simulink model "AOM"  (R2023a)
settings: Solver=ode4  StartTime=0.0  StopTime=4  FixedStep=0.001  RelTol=1e-3
values from neighbouring files (symbols this model uses):
  trajectory = readmatrix('test.csv')    [actor_critic.m]
undefined symbols (not defined in the file or in its folder): dot_X0, X0
libraries: rllib x1
settings Model: Creator=Ali  LastModifiedBy=Ali

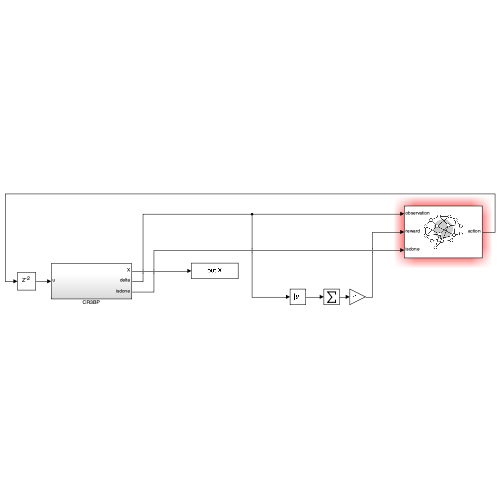
[thumbnail: Simulink's stored preview of the top-level diagram]
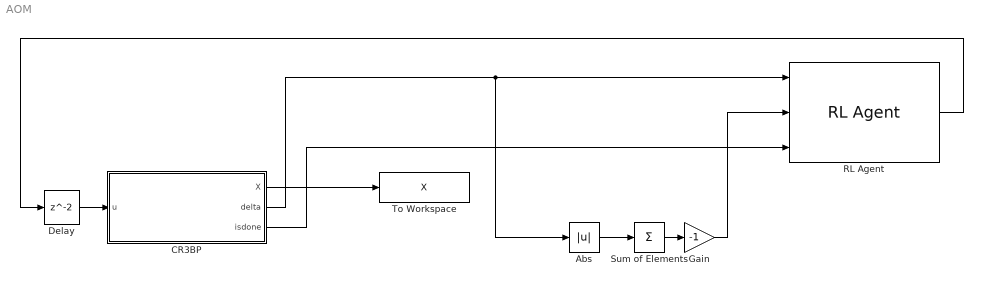
== system AOM ==
  Abs : Abs  SaturateOnIntegerOverflow=off
  CR3BP : Subsystem
  Delay : Delay
  Gain : Gain  Gain=-1
  RL Agent : rllib/RL Agent  Agent=agentObj  ExternalActionAsInput=off  ProvideLastAction=off  ProvideCumRwd=off  TreatAsDirectFeedthrough=on  UseStrictObservationDataTypes=off
  Sum of Elements : Sum  Inputs=+
  To Workspace : ToWorkspace  VariableName=X  SaveFormat=Timeseries  SampleTime=-1
  wires:
  CR3BP/1(X) -> To Workspace/1
  CR3BP/3(isdone) -> RL Agent/3
  RL Agent/1 -> Delay/1
  Delay/1 -> CR3BP/1(u)
  CR3BP/2(delta) -> Abs/1, RL Agent/1
  Abs/1 -> Sum of Elements/1
  Sum of Elements/1 -> Gain/1
  Gain/1 -> RL Agent/2

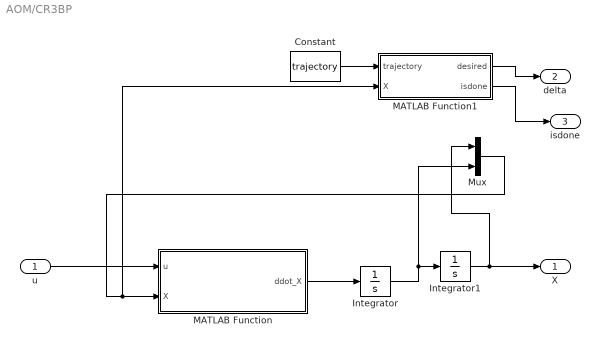
== system AOM/CR3BP ==
  u : Inport
  Constant : Constant  Value=trajectory
  Integrator : Integrator  InitialCondition=dot_X0
  Integrator1 : Integrator  InitialCondition=X0
  MATLAB Function : MATLAB Function  TreatAsAtomicUnit=on
  MATLAB Function1 : MATLAB Function  TreatAsAtomicUnit=on
  Mux : Mux  Inputs=2
  X : Outport
  delta : Outport  Port=2
  isdone : Outport  Port=3
  wires:
  u/1 -> MATLAB Function/1(u)
  Integrator1/1 -> Mux/1, X/1
  Integrator/1 -> Mux/2, Integrator1/1
  MATLAB Function/1(ddot_X) -> Integrator/1
  Mux/1 -> MATLAB Function1/2(X), MATLAB Function/2(X)
  Constant/1 -> MATLAB Function1/1(trajectory)
  MATLAB Function1/1(desired) -> delta/1
  MATLAB Function1/2(isdone) -> isdone/1

== matlab function AOM/CR3BP/MATLAB Function1 ==
  data: trajectory input; desired output size=[2, 1]; X input; isdone output
function [desired, isdone] = fcn(trajectory, X)



xy = X(1:2);
dist = sum((trajectory(:, 1:2) - xy).^2);
dist = dist';
index = dist==min(dist);
answer = trajectory(:, index);

desired = reshape(answer, [2, 1]) - reshape(xy, [2, 1]);

isdone = false;
if sum((xy - trajectory(end, 1:2)).^2) <= 0.01
    isdone = true;
end

== matlab function AOM/CR3BP/MATLAB Function ==
  data: u input; ddot_X output; X input
function ddot_X = fcn(u, X)

mu = 0.012277471;

a_x = u(1);
a_y = u(2);

% Positions
x = X(1);
y = X(2);
z = 0;
% Velocities
xdot = X(3);
ydot = X(4);

% distances from particle to primaries
r1 = sqrt((x+mu)^2 + y^2 + z^2); 
r2 = sqrt((x-1+mu)^2 + y^2 + z^2); 

% Accelerations 
xddot = 2*ydot + x -(1-mu)*((x+mu)/(r1^3)) - mu*(x-1+mu)/(r2^3) + a_x;
yddot = -2*xdot + y - (1-mu)*(y/(r1^3)) - mu*(y)/(r2^3) + a_y;

ddot_X = [xddot; yddot];
